simulink model "Fig1model"  (R2021a)
settings: Solver=VariableStepAuto  StartTime=0.0  StopTime=15000  FixedStep=.01  MaxStep=.0098  RelTol=1e-3
StartFcn:
  | disp('© 2025 Alireza Alemi. All rights reserved.');
values from neighbouring files (symbols this model uses):
  amplitSin = .004    (= 0.004)    [mainFig1.m]
  eta1 = .01    (= 0.01)    [mainFig1.m]
  eta2 = 0    [mainFig1.m]
  omega_nUnstb = .1    (= 0.1)    [mainFig1.m]
  omega_sd = 0.2    [mainFig1.m]
  perturbCASE = 2    [mainFig1.m]
  seed = 3    [mainFig1.m]    (also in mainFig4_rel.m = 2)
  StopTime = StopTime/10    (= 1500)    [mainFig1.m]
libraries: dspsrcs4 x1
Description:
  | %-----------------------------------------------------------------------------
  | % Copyright (c) 2025 Alireza Alemi
  | % Licensed under the Non-Commercial License (for non-commercial use only).
  | % For commercial use, a separate commercial license must be obtained.
  | % For more information, contact alireza.alemi@gmail.com
  | %-----------------------------------------------------------------------------
settings Model: Creator=alemi  LastModifiedBy=alemi
settings SolverCC: ShapePreserveControl=EnableAll

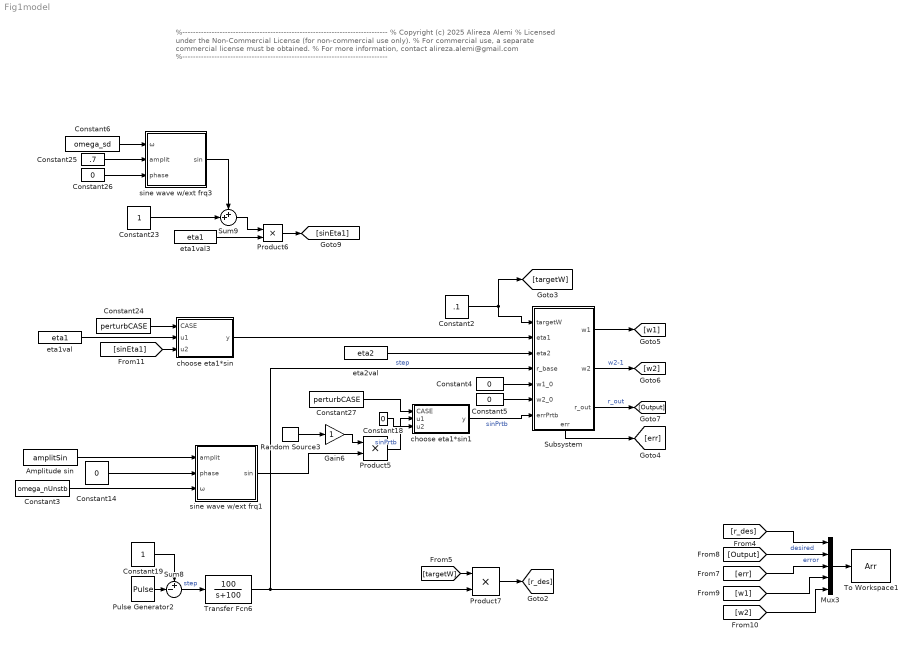
== system Fig1model ==
  note: %-----------------------------------------------------------------------------
      | % Copyright (c) 2025 Alireza Alemi
      | % Licensed under the Non-Commercial License (for non-commercial use only).
      | % For commercial use, a separate commercial license must be obtained.
      | % For more information, contact alireza.alemi@gmail.com
      | %-----------------------------------------------------------------------------
  Amplitude sin : Constant  Value=amplitSin
  Constant{4..5,14,18,26} (5 alike) : Constant  Value=0
  Constant19 : Constant
  Constant2 : Constant  Value=.1
  Constant23 : Constant
  Constant24 : Constant  Value=perturbCASE
  Constant25 : Constant  Value=.7
  Constant27 : Constant  Value=perturbCASE
  Constant3 : Constant  Value=omega_nUnstb
  Constant6 : Constant  Value=omega_sd
  Gain6 : Gain
  Mux3 : Mux  Inputs=5
  Product5 : Product
  Product6 : Product
  Product7 : Product
  Pulse Generator2 : DiscretePulseGenerator  PulseType=Time based  Period=StopTime+.1  PulseWidth=2
  Random Source3 : dspsrcs4/Random Source  SrcType=Uniform  NormMethod=Ziggurat  CltLength=12  MinVal=0  MaxVal=1  MeanVal=0  VarVal=1  RepMode=Specify seed  rawSeed=seed+1  IsInherit=off  SampMode=Discrete  SampTime=100  SampFrame=1  DataType=Double  OutComplex=Real  OutputFrames=off
  Subsystem : Subsystem  Description=|
      | %-----------------------------------------------------------------------------
      | % Copyright (c) 2025 Alireza Alemi 
      | % Licensed under the Non-Commercial License (for non-commercial use only).
      | % For commercial use, a separate commercial license must be obtained.
      | % For more information, contact alireza.alemi@gmail.com
      | %-----------------------------------------------------------------------------
      settings: PortSchema="{\"entries\":[{\"content\":{\"sides\":[{\"content\":{\"connectorIds\":[\"In1\",\"In2\",\"In3\",\"In4\",\"In5\",\"In6\",\"In7\"]},\"type\":\"ConnectorPlacement.EquallySpacedRectSide\",\"uuid\":\"f4103d7f-83fd-4af7-b9e6-e4c3830d16fd\"},{\"content\":{\"connectorIds\":[\"Out1\",\"Out2\",\"Out3\"],\"side\":\"RIGHT\"},\"type\":\"ConnectorPlacement.EquallySpacedRectSide\",\"uuid\":\"89738b27-e148-48c9-aa81-4b16f7796127\"},{\"content\":{\"connectorIds\":[],\"side\":\"TOP\"},\"type\":\"ConnectorPlacement.EquallySpacedRectSide\",\"uuid\":\"a85b5c3c-be84-4add-b485-c641517a9b08\"},{\"content\":{\"connectorIds\":[\"Out4\"],\"side\":\"BOTTOM\"},\"type\":\"ConnectorPlacement.EquallySpacedRectSide\",\"uuid\":\"6c5c5169-fb3e-4152-9cab-afb906ac9f65\"}]},\"type\":\"ConnectorPlacement.EquallySpacedConnector\",\"uuid\":\"8f7f0c07-3153-4818-b2c3-45fb0ad6ae46\"}],\"packageUris\":[\"http://schema.mathworks.com/mf0/Connector/R2020b\"],\"version\":\"1.0\"}"
  Sum8 : Sum  Inputs=+-|
  Sum9 : Sum  Inputs=++|
  To Workspace1 : ToWorkspace  VariableName=Arr  SaveFormat=Timeseries  SampleTime=-1
      settings: Save2DSignal=2-D array (concatenate along first dimension)
  Transfer Fcn6 : TransferFcn  Numerator=[100]  Denominator=[1 100]
  choose eta1*sin : MATLAB Function  TreatAsAtomicUnit=on
  choose eta1*sin1 : MATLAB Function  TreatAsAtomicUnit=on
  eta1val : Constant  Value=eta1
  eta1val3 : Constant  Value=eta1
  eta2val : Constant  Value=eta2
  sine wave w/ext frq1 : Subsystem
  sine wave w/ext frq3 : Subsystem
  wires:
  Subsystem/1(w1) -> [w1]
  eta1val/1 -> choose eta1*sin/2(u1)
  Constant4/1 -> Subsystem/5(w1_0)
  Subsystem/3(r_out) -> [Output]  "r_out"
  Constant2/1 -> [targetW], Subsystem/1(targetW)
  Constant5/1 -> Subsystem/6(w2_0)
  choose eta1*sin1/1(y) -> Subsystem/7(errPrtb)  "sinPrtb"
  Subsystem/2(w2) -> [w2]  "w2-1"
  sine wave w/ext frq1/1(sin) -> Product5/2
  Constant14/1 -> sine wave w/ext frq1/2(phase)
  Subsystem/4(err) -> [err]
  Constant3/1 -> sine wave w/ext frq1/3(ω)
  eta2val/1 -> Subsystem/3(eta2)
  Random Source3/1 -> Gain6/1
  Gain6/1 -> Product5/1
  [targetW] -> Product7/1
  Product7/1 -> [r_des]
  [r_des] -> Mux3/1  "desired"
  Mux3/1 -> To Workspace1/1
  [Output] -> Mux3/2
  [w2] -> Mux3/5
  [w1] -> Mux3/4
  [err] -> Mux3/3  "error"
  Pulse Generator2/1 -> Sum8/2
  Constant19/1 -> Sum8/1
  Transfer Fcn6/1 -> Product7/2, Subsystem/4(r_base)  "step"
  Sum8/1 -> Transfer Fcn6/1  "step"
  Constant23/1 -> Sum9/2
  Sum9/1 -> Product6/1
  Product6/1 -> [sinEta1]
  eta1val3/1 -> Product6/2
  sine wave w/ext frq3/1(sin) -> Sum9/1
  choose eta1*sin/1(y) -> Subsystem/2(eta1)
  Constant24/1 -> choose eta1*sin/1(CASE)
  Constant25/1 -> sine wave w/ext frq3/2(amplit)
  Constant26/1 -> sine wave w/ext frq3/3(phase)
  Constant6/1 -> sine wave w/ext frq3/1(ω)
  [sinEta1] -> choose eta1*sin/3(u2)
  Constant27/1 -> choose eta1*sin1/1(CASE)
  Product5/1 -> choose eta1*sin1/2(u1)  "sinPrtb"
  Constant18/1 -> choose eta1*sin1/3(u2)
  Amplitude sin/1 -> sine wave w/ext frq1/1(amplit)

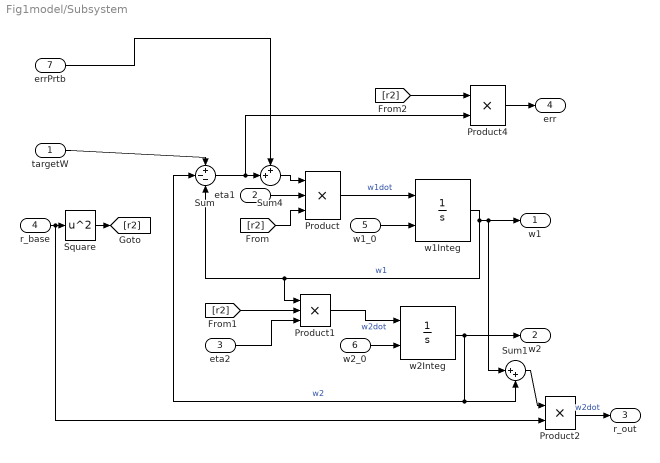
== system Fig1model/Subsystem ==
  targetW : Inport
  eta1 : Inport  Port=2
  eta2 : Inport  Port=3
  r_base : Inport  Port=4
  w1_0 : Inport  Port=5
  w2_0 : Inport  Port=6
  errPrtb : Inport  Port=7
  Product : Product  Inputs=3
  Product1 : Product  Inputs=3
  Product2 : Product
  Product4 : Product
  Square : Math  Operator=square  SaturateOnIntegerOverflow=on
  Sum : Sum  Inputs=+--
  Sum1 : Sum  Inputs=|++
  Sum4 : Sum  Inputs=++|
  w1Integ : Integrator  InitialConditionSource=external
  w2Integ : Integrator  InitialConditionSource=external
  w1 : Outport
  w2 : Outport  Port=2
  r_out : Outport  Port=3
  err : Outport  Port=4
  wires:
  eta2/1 -> Product1/3
  Sum4/1 -> Product/1
  Product1/1 -> w2Integ/1  "w2dot"
  r_base/1 -> Product2/2, Square/1
  w1Integ/1 -> Sum/3, Product1/1, w1/1, Sum1/1  "w1"
  w1_0/1 -> w1Integ/2
  w2_0/1 -> w2Integ/2
  w2Integ/1 -> w2/1, Sum1/2, Sum/2  "w2"
  [r2] -> Product/3
  [r2] -> Product1/2
  Square/1 -> [r2]
  eta1/1 -> Product/2
  targetW/1 -> Sum/1
  Sum1/1 -> Product2/1
  Product2/1 -> r_out/1  "w2dot"
  Product/1 -> w1Integ/1  "w1dot"
  Sum/1 -> Product4/2, Sum4/2
  errPrtb/1 -> Sum4/1
  Product4/1 -> err/1
  [r2] -> Product4/1

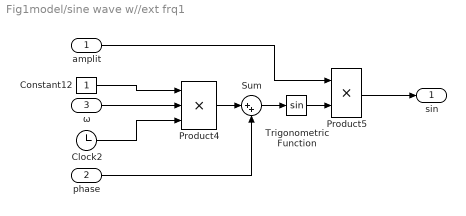
== system Fig1model/sine wave w//ext frq1 ==
  amplit : Inport
  phase : Inport  Port=2
  ω : Inport  Port=3
  Clock2 : Clock
  Constant12 : Constant
  Product4 : Product  Inputs=3
  Product5 : Product
  Sum : Sum  Inputs=|++
  Trigonometric Function : Trigonometry
  sin : Outport
  wires:
  amplit/1 -> Product5/1
  Product4/1 -> Sum/1
  Constant12/1 -> Product4/1
  ω/1 -> Product4/2
  Product5/1 -> sin/1
  Clock2/1 -> Product4/3
  Trigonometric Function/1 -> Product5/2
  phase/1 -> Sum/2
  Sum/1 -> Trigonometric Function/1

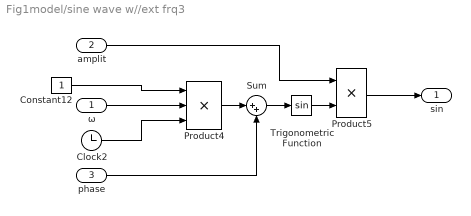
== system Fig1model/sine wave w//ext frq3 ==
  ω : Inport
  amplit : Inport  Port=2
  phase : Inport  Port=3
  Clock2 : Clock
  Constant12 : Constant
  Product4 : Product  Inputs=3
  Product5 : Product
  Sum : Sum  Inputs=|++
  Trigonometric Function : Trigonometry
  sin : Outport
  wires:
  amplit/1 -> Product5/1
  Product4/1 -> Sum/1
  Constant12/1 -> Product4/1
  ω/1 -> Product4/2
  Product5/1 -> sin/1
  Clock2/1 -> Product4/3
  Trigonometric Function/1 -> Product5/2
  phase/1 -> Sum/2
  Sum/1 -> Trigonometric Function/1

== matlab function Fig1model/choose eta1*sin1 ==
  data: CASE input; y output; u1 input; u2 input
function y = fcn(CASE, u1, u2)
    y=u1;
    if CASE==1
        y = u1;
    elseif CASE==2
        y = u2;
    else
        error('valueError')
    end
end

== matlab function Fig1model/choose eta1*sin ==
  data: CASE input; y output; u1 input; u2 input
function y = fcn(CASE, u1, u2)
    y=u1;
    if CASE==1
        y = u1;
    elseif CASE==2
        y = u2;
    else
        error('valueError')
    end
end
